simulink model "lin_val"  (R2023b)
settings: Solver=VariableStepAuto  StartTime=0.0  StopTime=90  MaxStep=1e-3  RelTol=1e-6
values from neighbouring files (symbols this model uses):
  linsysROV = linearize_ROV(ROV, Velocity, Position, V0, Reduced)    [CreateGramianROV.m]    (also in Linearization_validation.m = linearize_ROV(ROV,v_init', eta_init', 0); ROV_simulation_init.m = linearize_ROV(ROV,v_init', eta_init', 0))
  ROV = initializeModelMatrices(m,I,COG,l,w,h,Thrusters)    [CreateGramianROV.m]    (also in CreateROVLin.m = initializeModelMatrices(m, I, COB, dim, BlueROVHeavy); Eigenvalue_tracking.m = initializeModelMatrices(m, I, COB,dim,0); Linearization_validation.m = initializeModelMatrices(m, I, COB,dim,0); ROV_simulation_init.m = initializeModelMatrices(m, Inertia, COB, dim, BlueROVHeavy))
  u_diff = (ROV.T'/(ROV.T*ROV.T'))*(F_diff)    [Linearization_validation.m]
  v_init = [1 0 0 0 0 0]    [Linearization_validation.m]    (also in ROV_simulation_init.m = [omega omega z_rate 0 0 omega])
settings Model: Creator=Tomas  LastModifiedBy=Ottol

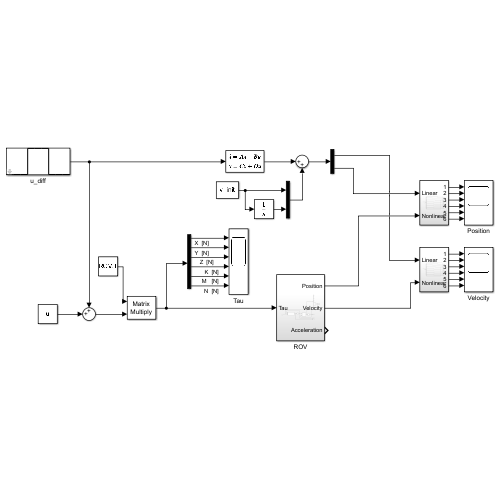
[thumbnail: Simulink's stored preview of the top-level diagram]
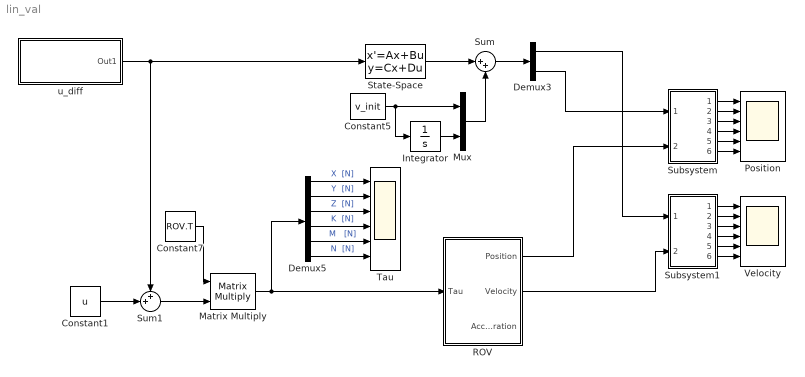
== system lin_val ==
  Constant1 : Constant  Value=u
  Constant5 : Constant  Value=v_init
  Constant7 : Constant  Value=ROV.T
  Demux3 : Demux  Outputs=2
  Demux5 : Demux  Outputs=6
  Integrator : Integrator
  Matrix Multiply : Product  Multiplication=Matrix(*)
  Mux : Mux  Inputs=2
  Position : Scope  NumInputPorts=6
  ROV : Subsystem
  State-Space : StateSpace  A=linsysROV.A  B=linsysROV.B  C=linsysROV.C  D=linsysROV.D  InitialCondition=zeros(1,12)
  Subsystem : Subsystem
  Subsystem1 : Subsystem
  Sum : Sum  Inputs=|++
  Sum1 : Sum  Inputs=++|
  Tau : Scope  NumInputPorts=6
  Velocity : Scope  NumInputPorts=6
  u_diff : Subsystem  mask{Step_time_1=5, Step_time_2=25, Init_val=0, New_val=u_diff}
      mask prompts: Step_time_1 "Step time 1:"; Step_time_2 "Step time 2:"; Init_val "Inital Value:"; New_val "New Value:"
      mask Display: plot([1 2 3 4 4 5 6 7 7 8 9 10],[0 0 0 0 1 1 1 1 0 0 0 0]);
  wires:
  Constant7/1 -> Matrix Multiply/1
  State-Space/1 -> Sum/1
  Constant1/1 -> Sum1/2
  Sum/1 -> Demux3/1
  Demux5/3 -> Tau/3  "Z  [N]"
  Demux5/4 -> Tau/4  "K  [N]"
  Demux5/5 -> Tau/5  "M   [N]"
  Demux5/6 -> Tau/6  "N  [N]"
  Demux5/2 -> Tau/2  "Y  [N]"
  Demux5/1 -> Tau/1  "X  [N]"
  Subsystem/6(Out6) -> Position/6
  Subsystem/1(Out1) -> Position/1
  Subsystem/2(Out2) -> Position/2
  Subsystem/5(Out5) -> Position/5
  Subsystem/4(Out4) -> Position/4
  Subsystem/3(Out3) -> Position/3
  Subsystem1/1(Out1) -> Velocity/1
  Subsystem1/5(Out5) -> Velocity/5
  Subsystem1/2(Out2) -> Velocity/2
  Subsystem1/4(Out4) -> Velocity/4
  Subsystem1/3(Out3) -> Velocity/3
  Subsystem1/6(Out6) -> Velocity/6
  Demux3/2 -> Subsystem/1(Linear)
  ROV/1(Position) -> Subsystem/2(Nonlinear)
  ROV/2(Velocity) -> Subsystem1/2(Nonlinear)
  Demux3/1 -> Subsystem1/1(Linear)
  Matrix Multiply/1 -> ROV/1(Tau), Demux5/1
  u_diff/1(Out1) -> State-Space/1, Sum1/1
  Sum1/1 -> Matrix Multiply/2
  Integrator/1 -> Mux/2
  Constant5/1 -> Mux/1, Integrator/1
  Mux/1 -> Sum/2

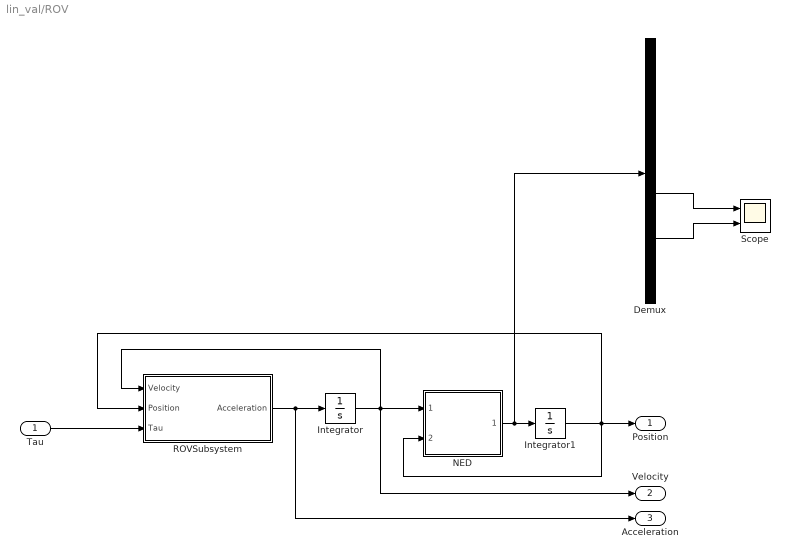
== system lin_val/ROV ==
  Tau : Inport
  Demux : Demux  Outputs=6
  Integrator : Integrator  InitialCondition=v_init'
  Integrator1 : Integrator  InitialCondition=eta_init'
  NED : Subsystem
  ROVSubsystem : Subsystem
  Scope : Scope  NumInputPorts=2
  Position : Outport
  Velocity : Outport  Port=2
  Acceleration : Outport  Port=3
  wires:
  Integrator/1 -> Velocity/1, NED/1(velocity), ROVSubsystem/1(Velocity)
  Integrator1/1 -> Position/1, ROVSubsystem/2(Position), NED/2(position_NED)
  ROVSubsystem/1(Acceleration) -> Acceleration/1, Integrator/1
  Tau/1 -> ROVSubsystem/3(Tau)
  NED/1(Velocity_NED) -> Demux/1, Integrator1/1
  Demux/4 -> Scope/1
  Demux/5 -> Scope/2

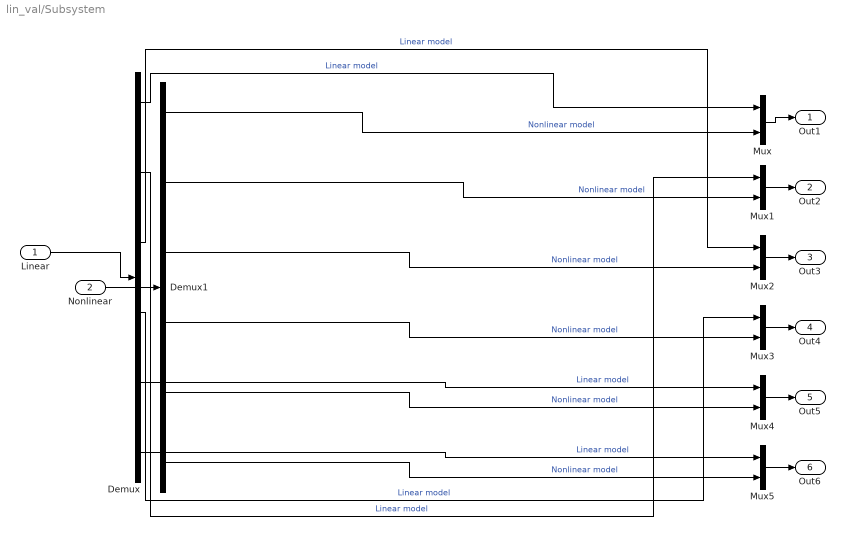
== system lin_val/Subsystem ==
  Linear : Inport
  Nonlinear : Inport  Port=2
  Demux : Demux  Outputs=6
  Demux1 : Demux  Outputs=6
  Mux{,1..5} (6 alike) : Mux  Inputs=2
  Out1 : Outport
  Out2 : Outport  Port=2
  Out3 : Outport  Port=3
  Out4 : Outport  Port=4
  Out5 : Outport  Port=5
  Out6 : Outport  Port=6
  wires:
  Demux/4 -> Mux3/1  "Linear model"
  Demux/5 -> Mux4/1  "Linear model"
  Demux/6 -> Mux5/1  "Linear model"
  Demux/1 -> Mux/1  "Linear model"
  Demux/2 -> Mux1/1  "Linear model"
  Linear/1 -> Demux/1
  Demux/3 -> Mux2/1  "Linear model"
  Mux/1 -> Out1/1
  Mux1/1 -> Out2/1
  Mux2/1 -> Out3/1
  Mux5/1 -> Out6/1
  Mux4/1 -> Out5/1
  Mux3/1 -> Out4/1
  Nonlinear/1 -> Demux1/1
  Demux1/1 -> Mux/2  "Nonlinear model"
  Demux1/2 -> Mux1/2  "Nonlinear model"
  Demux1/3 -> Mux2/2  "Nonlinear model"
  Demux1/4 -> Mux3/2  "Nonlinear model"
  Demux1/5 -> Mux4/2  "Nonlinear model"
  Demux1/6 -> Mux5/2  "Nonlinear model"

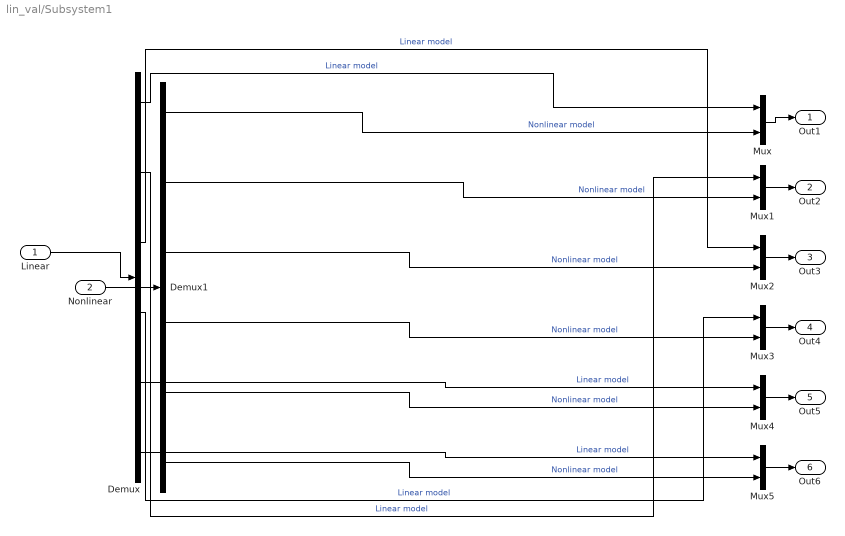
== system lin_val/Subsystem1 ==
  Linear : Inport
  Nonlinear : Inport  Port=2
  Demux : Demux  Outputs=6
  Demux1 : Demux  Outputs=6
  Mux{,1..5} (6 alike) : Mux  Inputs=2
  Out1 : Outport
  Out2 : Outport  Port=2
  Out3 : Outport  Port=3
  Out4 : Outport  Port=4
  Out5 : Outport  Port=5
  Out6 : Outport  Port=6
  wires:
  Demux/4 -> Mux3/1  "Linear model"
  Demux/5 -> Mux4/1  "Linear model"
  Demux/6 -> Mux5/1  "Linear model"
  Demux/1 -> Mux/1  "Linear model"
  Demux/2 -> Mux1/1  "Linear model"
  Linear/1 -> Demux/1
  Demux/3 -> Mux2/1  "Linear model"
  Mux/1 -> Out1/1
  Mux1/1 -> Out2/1
  Mux2/1 -> Out3/1
  Mux5/1 -> Out6/1
  Mux4/1 -> Out5/1
  Mux3/1 -> Out4/1
  Nonlinear/1 -> Demux1/1
  Demux1/1 -> Mux/2  "Nonlinear model"
  Demux1/2 -> Mux1/2  "Nonlinear model"
  Demux1/3 -> Mux2/2  "Nonlinear model"
  Demux1/4 -> Mux3/2  "Nonlinear model"
  Demux1/5 -> Mux4/2  "Nonlinear model"
  Demux1/6 -> Mux5/2  "Nonlinear model"

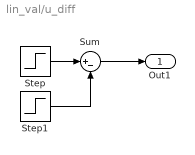
== system lin_val/u_diff ==
  Step : Step  Time=Step_time_1  Before=Init_val  After=New_val  SampleTime=0
  Step1 : Step  Time=Step_time_2  After=New_val  SampleTime=0
  Sum : Sum  Inputs=|+-
  Out1 : Outport
  wires:
  Sum/1 -> Out1/1
  Step/1 -> Sum/1
  Step1/1 -> Sum/2

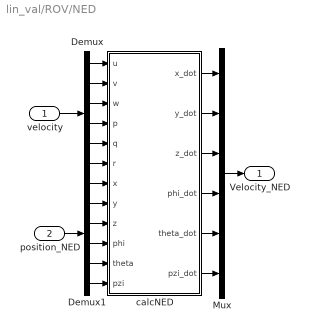
== system lin_val/ROV/NED ==
  velocity : Inport
  position_NED : Inport  Port=2
  Demux : Demux  Outputs=6
  Demux1 : Demux  Outputs=6
  Mux : Mux  Inputs=6
  calcNED : MATLAB Function  TreatAsAtomicUnit=on
  Velocity_NED : Outport
  wires:
  calcNED/2(y_dot) -> Mux/2
  Demux1/5 -> calcNED/11(theta)
  Demux1/4 -> calcNED/10(phi)
  calcNED/1(x_dot) -> Mux/1
  calcNED/3(z_dot) -> Mux/3
  calcNED/5(theta_dot) -> Mux/5
  Demux1/3 -> calcNED/9(z)
  calcNED/4(phi_dot) -> Mux/4
  calcNED/6(pzi_dot) -> Mux/6
  Demux1/2 -> calcNED/8(y)
  Demux/4 -> calcNED/4(p)
  Demux1/6 -> calcNED/12(pzi)
  Demux1/1 -> calcNED/7(x)
  velocity/1 -> Demux/1
  Demux/2 -> calcNED/2(v)
  Demux/1 -> calcNED/1(u)
  Demux/5 -> calcNED/5(q)
  Demux/6 -> calcNED/6(r)
  Demux/3 -> calcNED/3(w)
  position_NED/1 -> Demux1/1
  Mux/1 -> Velocity_NED/1

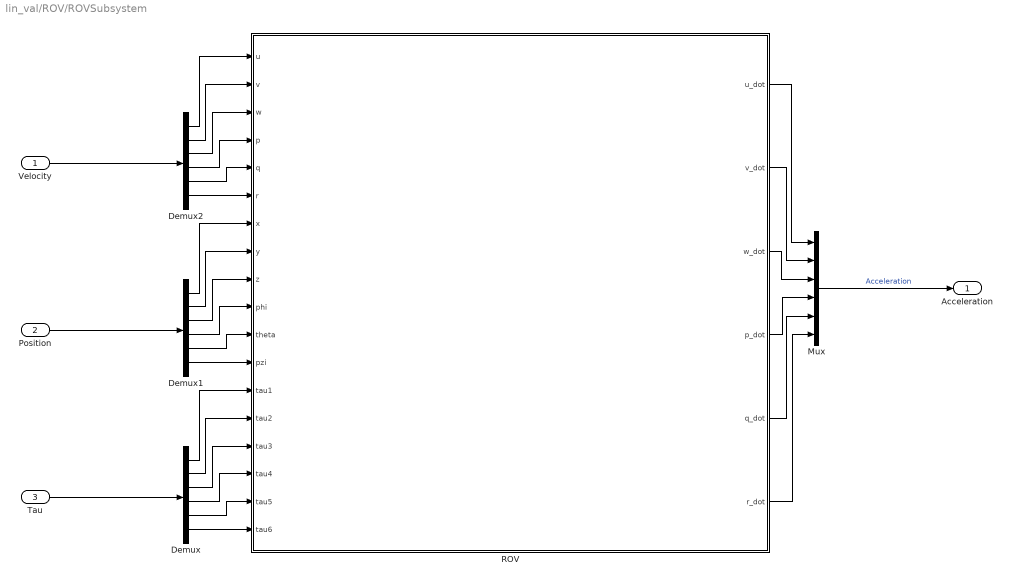
== system lin_val/ROV/ROVSubsystem ==
  Velocity : Inport
  Position : Inport  Port=2
  Tau : Inport  Port=3
  Demux : Demux  Outputs=6
  Demux1 : Demux  Outputs=6
  Demux2 : Demux  Outputs=6
  Mux : Mux  Inputs=6
  ROV : MATLAB Function  TreatAsAtomicUnit=on
  Acceleration : Outport
  wires:
  Demux1/1 -> ROV/7(x)
  Demux2/3 -> ROV/3(w)
  ROV/6(r_dot) -> Mux/6
  Demux/2 -> ROV/14(tau2)
  Mux/1 -> Acceleration/1  "Acceleration"
  Demux/4 -> ROV/16(tau4)
  Tau/1 -> Demux/1
  ROV/3(w_dot) -> Mux/3
  ROV/4(p_dot) -> Mux/4
  Demux/6 -> ROV/18(tau6)
  Demux1/2 -> ROV/8(y)
  ROV/1(u_dot) -> Mux/1
  Demux1/3 -> ROV/9(z)
  Demux1/5 -> ROV/11(theta)
  Demux2/6 -> ROV/6(r)
  Demux/1 -> ROV/13(tau1)
  Demux2/4 -> ROV/4(p)
  Velocity/1 -> Demux2/1
  Demux2/5 -> ROV/5(q)
  Demux2/1 -> ROV/1(u)
  Demux/5 -> ROV/17(tau5)
  ROV/5(q_dot) -> Mux/5
  Demux/3 -> ROV/15(tau3)
  Demux1/6 -> ROV/12(pzi)
  Demux1/4 -> ROV/10(phi)
  Demux2/2 -> ROV/2(v)
  ROV/2(v_dot) -> Mux/2
  Position/1 -> Demux1/1

== matlab function lin_val/ROV/NED/calcNED ==
  data: u input; x_dot output; v input; w input; p input; q input; r input; x input; y input; z input; phi input; theta input; pzi input; y_dot output; z_dot output; phi_dot output; theta_dot output; pzi_dot output
function [x_dot,y_dot,z_dot,phi_dot,theta_dot,pzi_dot] = calcNED(u,v,w,p,q,r,x,y,z,phi,theta,pzi)
%#codegen

%    This function was generated by the Symbolic Math Toolbox version 23.2.
%    12-Jun-2024 23:09:41

% u = complex(u);  % if required to enforce complex operations
% v = complex(v);  % if required to enforce complex operations
% w = complex(w);  % if required to enforce complex operations
% p = complex(p);  % if required to enforce complex operations
% q = complex(q);  % if required to enforce complex operations
% r = complex(r);  % if required to enforce complex operations
% x = complex(x);  % if required to enforce complex operations
% y = complex(y);  % if required to enforce complex operations
% z = complex(z);  % if required to enforce complex operations
% phi = complex(phi);  % if required to enforce complex operations
% theta = complex(theta);  % if required to enforce complex operations
% pzi = complex(pzi);  % if required to enforce complex operations
t2 = cos(phi);
t3 = cos(pzi);
t4 = cos(theta);
t5 = sin(phi);
t6 = sin(pzi);
t7 = sin(theta);
x_dot = -v.*(t2.*t6-t3.*t5.*t7)+w.*(t5.*t6+t2.*t3.*t7)+t3.*t4.*u;
if nargout > 1
    y_dot = v.*(t2.*t3+t5.*t6.*t7)-w.*(t3.*t5-t2.*t6.*t7)+t4.*t6.*u;
end
if nargout > 2
    z_dot = -t7.*u+t4.*t5.*v+t2.*t4.*w;
end
if nargout > 3
    t8 = tan(theta);
    phi_dot = p+q.*t5.*t8+r.*t2.*t8;
end
if nargout > 4
    theta_dot = q.*t2-r.*t5;
end
if nargout > 5
    t9 = 1.0./t4;
    pzi_dot = q.*t5.*t9+r.*t2.*t9;
end
end

== matlab function lin_val/ROV/ROVSubsystem/ROV ==
  data: u input; u_dot output; v input; w input; p input; q input; r input; x input; y input; z input; phi input; theta input; pzi input; tau1 input; tau2 input; tau3 input; tau4 input; tau5 input; tau6 input; v_dot output; w_dot output; p_dot output; q_dot output; r_dot output
function [u_dot,v_dot,w_dot,p_dot,q_dot,r_dot] = ROV(u,v,w,p,q,r,x,y,z,phi,theta,pzi,tau1,tau2,tau3,tau4,tau5,tau6)
%#codegen

%    This function was generated by the Symbolic Math Toolbox version 23.2.
%    12-Jun-2024 23:09:41

% u = complex(u);  % if required to enforce complex operations
% v = complex(v);  % if required to enforce complex operations
% w = complex(w);  % if required to enforce complex operations
% p = complex(p);  % if required to enforce complex operations
% q = complex(q);  % if required to enforce complex operations
% r = complex(r);  % if required to enforce complex operations
% x = complex(x);  % if required to enforce complex operations
% y = complex(y);  % if required to enforce complex operations
% z = complex(z);  % if required to enforce complex operations
% phi = complex(phi);  % if required to enforce complex operations
% theta = complex(theta);  % if required to enforce complex operations
% pzi = complex(pzi);  % if required to enforce complex operations
% tau1 = complex(tau1);  % if required to enforce complex operations
% tau2 = complex(tau2);  % if required to enforce complex operations
% tau3 = complex(tau3);  % if required to enforce complex operations
% tau4 = complex(tau4);  % if required to enforce complex operations
% tau5 = complex(tau5);  % if required to enforce complex operations
% tau6 = complex(tau6);  % if required to enforce complex operations
u_dot = tau1.*2.645957976303975e-2-u.*3.531457518244686e-1-q.*w.*1.032231117827961+r.*v.*8.009610694239536e-1-u.*abs(u).*2.207160948902929;
if nargout > 1
    v_dot = tau2.*3.303478879700023e-2-v.*2.936116807508284e-1+p.*w.*1.288740685699412-r.*u.*1.24850013087302-v.*abs(v).*1.835073004692678;
end
if nargout > 2
    w_dot = tau3.*2.563338704486693e-2-w.*4.583524343112879e-1-p.*v.*7.759512919057802e-1+q.*u.*9.687752894954555e-1-w.*abs(w).*2.86470271444555;
end
if nargout > 3
    et1 = p.*(-4.371786229547364)+tau4.*1.52560031871831-cos(theta).*sin(phi).*7.645005934743983-q.*r.*3.44400732551688e-1-v.*w.*1.333451486058743e+1;
    et2 = p.*abs(p).*(-9.169266442461123e-1);
    p_dot = et1+et2;
end
if nargout > 4
    et3 = q.*(-5.04865589820956)+tau5.*2.034578627605437-sin(theta).*1.019557055141047e+1+p.*r.*1.256764688245948e-1+u.*w.*2.478374337910025;
    et4 = q.*abs(q).*(-6.844910552819897e-1);
    q_dot = et3+et4;
end
if nargout > 5
    r_dot = r.*(-5.514690819524503)+tau6.*1.394214122389249+p.*q.*2.286196223718177e-1+u.*v.*1.04878040543187e+1-r.*abs(r).*7.476755427021469e-1;
end
end
